simulink model "AC_Quadcopter_Simulation_Lyapnov_Hamilton_ITAE"  (R2015b)
settings: Solver=ode23  StartTime=0.0  StopTime=10  RelTol=1e-3
settings Model: Creator=HKJ  LastModifiedBy=HL

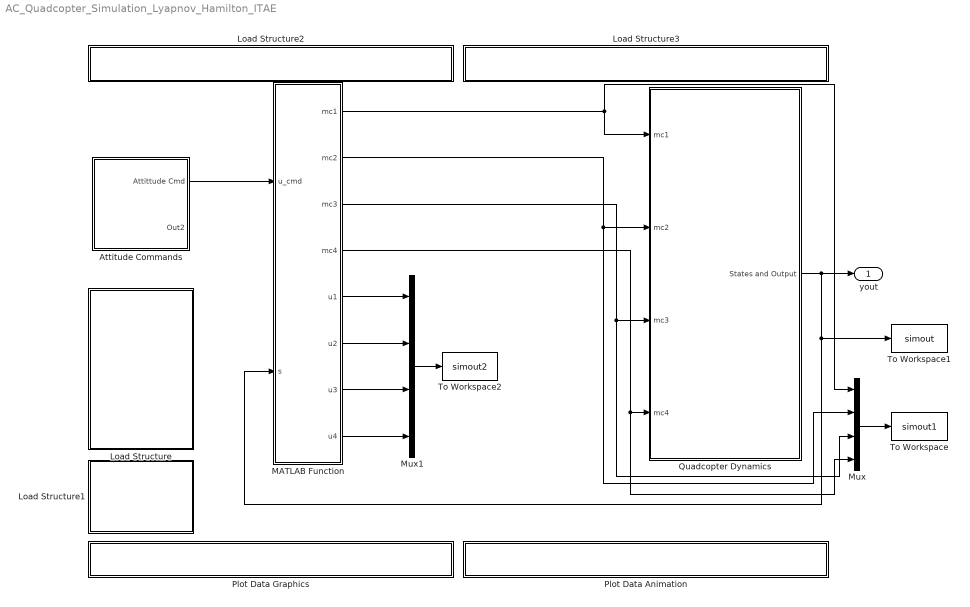
== system AC_Quadcopter_Simulation_Lyapnov_Hamilton_ITAE ==
  Attitude Commands : Subsystem
  Load Structure : Subsystem
      settings: OpenFcn=|
      | uiopen('load')
      | if (exist('IC')==1 && exist('quadModel')==1)
      | set_param(bdroot, 'SimulationCommand', 'update')
      | end
      mask Display: fprintf('LOAD:\nQuadcopter\nModel Or\nInitial\nConditions');
  Load Structure1 : Subsystem
      settings: OpenFcn=|
      | if (exist('IC')==1 && exist('quadModel')==1 && exist('yout') && exist('tout'))
      | saveSimResults()
      | else
      | msgbox('No Data To Save!')
      | end
      mask Display: fprintf('SAVE:\nSimulation\nResults');
  Load Structure2 : Subsystem
      settings: OpenFcn=|
      | if exist('GUI_Modeling') == 2,
      | run('GUI_Modeling')
      | 
      | else
      | 
      | msgbox('The desired GUI must be first added to MATLABs path.')
      | 
      | end
      mask Display: fprintf('OPEN GUI: Build New \n Model');
  Load Structure3 : Subsystem
      settings: OpenFcn=|
      | if exist('GUI_IC') == 2,
      | run('GUI_IC')
      | 
      | else
      | 
      | msgbox('The desired GUI must be first added to MATLABs path.')
      | 
      | end
      mask Display: fprintf('OPEN GUI: Create Initial \n Conditions');
  MATLAB Function : MATLAB Function  TreatAsAtomicUnit=on
  Mux : Mux
  Mux1 : Mux
  Plot Data Animation : Subsystem
      settings: OpenFcn=|
      | if exist('QuadAnim4') == 2,
      |     if exist('yout')
      | 	run('QuadAnim4');
      |     else
      |     msgbox('Simulation must be run before data can be plotted.');
      |     end
      | else                                                                          msgbox('The desired GUI must be first added to MATLABs path.')
      | end
      mask Display: fprintf('OPEN GUI: Flight Animation')
  Plot Data Graphics : Subsystem
      settings: OpenFcn=|
      | if exist('yout')
      | yout = evalin('base', 'yout');
      | tout = evalin('base', 'tout');
      | quadPlots(yout, tout)
      | else
      | msgbox('Simulation must be run before data can be plotted.')
      | end
      mask Display: fprintf('OPEN PLOT: State Data')
  Quadcopter Dynamics : Subsystem
  To Workspace : ToWorkspace  VariableName=simout1  SampleTime=-1
      settings: Save2DSignal=2-D array (concatenate along first dimension)
  To Workspace1 : ToWorkspace  VariableName=simout  SampleTime=-1
      settings: Save2DSignal=2-D array (concatenate along first dimension)
  To Workspace2 : ToWorkspace  VariableName=simout2  SampleTime=-1
      settings: Save2DSignal=2-D array (concatenate along first dimension)
  yout : Outport
  wires:
  Quadcopter Dynamics/1(States and Output) -> To Workspace1/1, MATLAB Function/2(s), yout/1
  MATLAB Function/1(mc1) -> Quadcopter Dynamics/1(mc1), Mux/1
  MATLAB Function/2(mc2) -> Quadcopter Dynamics/2(mc2), Mux/2
  MATLAB Function/3(mc3) -> Quadcopter Dynamics/3(mc3), Mux/3
  MATLAB Function/4(mc4) -> Quadcopter Dynamics/4(mc4), Mux/4
  Attitude Commands/1(Attittude Cmd) -> MATLAB Function/1(u_cmd)
  Mux/1 -> To Workspace/1
  Mux1/1 -> To Workspace2/1
  MATLAB Function/5(u1) -> Mux1/1
  MATLAB Function/6(u2) -> Mux1/2
  MATLAB Function/7(u3) -> Mux1/3
  MATLAB Function/8(u4) -> Mux1/4

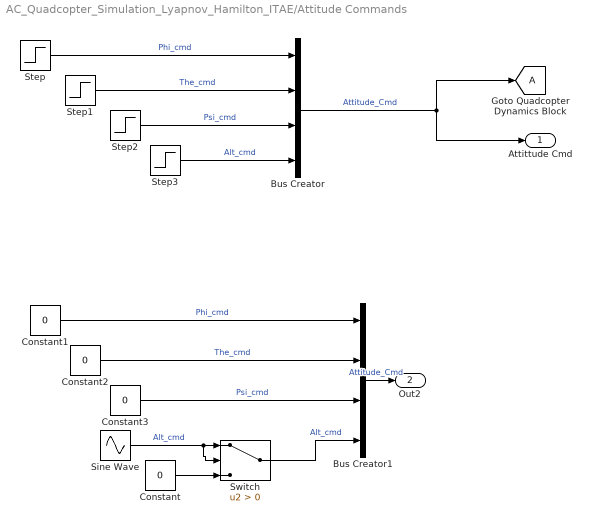
== system AC_Quadcopter_Simulation_Lyapnov_Hamilton_ITAE/Attitude Commands ==
  Bus Creator : BusCreator  Inputs=4
  Bus Creator1 : BusCreator  Inputs=4
  Constant{,1..3} (4 alike) : Constant  Value=0
  Sine Wave : Sin  Amplitude=10*0.3048  Frequency=0.2*3.1415
  Step : Step  Time=0  After=-15*pi/180  SampleTime=0
  Step1 : Step  Time=0  After=15*pi/180  SampleTime=0
  Step2 : Step  Time=0  After=15*pi/180  SampleTime=0
  Step3 : Step  Time=0  After=-1  SampleTime=0
  Switch : Switch  Criteria=u2 > Threshold
  Attittude Cmd : Outport
  Out2 : Outport  Port=2
  tag scope: A=global
  wires:
  Bus Creator/1 -> Attittude Cmd/1, [A]  "Attitude_Cmd"
  Step3/1 -> Bus Creator/4  "Alt_cmd"
  Step2/1 -> Bus Creator/3  "Psi_cmd"
  Step1/1 -> Bus Creator/2  "The_cmd"
  Step/1 -> Bus Creator/1  "Phi_cmd"
  Constant3/1 -> Bus Creator1/3  "Psi_cmd"
  Constant2/1 -> Bus Creator1/2  "The_cmd"
  Constant1/1 -> Bus Creator1/1  "Phi_cmd"
  Sine Wave/1 -> Switch/2, Switch/1  "Alt_cmd"
  Switch/1 -> Bus Creator1/4  "Alt_cmd"
  Constant/1 -> Switch/3
  Bus Creator1/1 -> Out2/1  "Attitude_Cmd"

== system AC_Quadcopter_Simulation_Lyapnov_Hamilton_ITAE/Load Structure ==

== system AC_Quadcopter_Simulation_Lyapnov_Hamilton_ITAE/Load Structure1 ==

== system AC_Quadcopter_Simulation_Lyapnov_Hamilton_ITAE/Load Structure2 ==

== system AC_Quadcopter_Simulation_Lyapnov_Hamilton_ITAE/Load Structure3 ==

== system AC_Quadcopter_Simulation_Lyapnov_Hamilton_ITAE/Plot Data Animation ==

== system AC_Quadcopter_Simulation_Lyapnov_Hamilton_ITAE/Plot Data Graphics ==

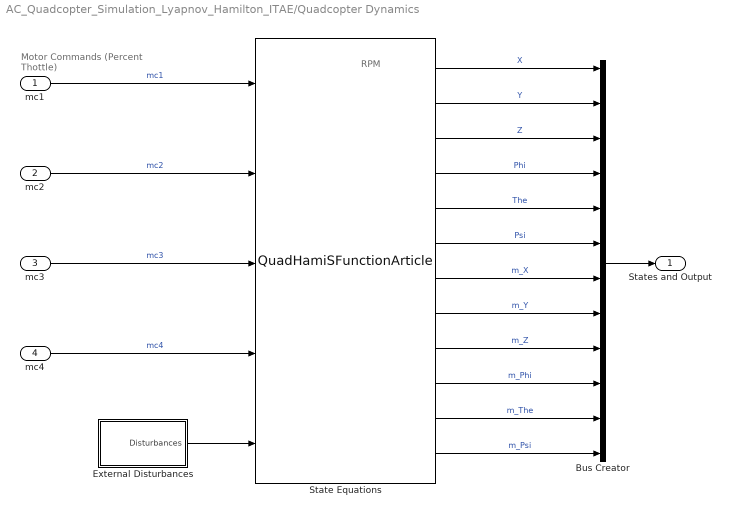
== system AC_Quadcopter_Simulation_Lyapnov_Hamilton_ITAE/Quadcopter Dynamics ==
  note: Motor Commands
      | (Percent Thottle)
  note: RPM
  mc1 : Inport
  mc2 : Inport  Port=2
  mc3 : Inport  Port=3
  mc4 : Inport  Port=4
  Bus Creator : BusCreator  Inputs='X','Y','Z','Phi','The','Psi','m_X','m_Y','m_Z','m_Phi','m_The','m_Psi'
  External Disturbances : Subsystem
  State Equations : M-S-Function  FunctionName=QuadHamiSFunctionArticle  Parameters=quadModel, IC
      mask Display:
      | port_label('input', 1, 'RPM1')
      | port_label('input', 2, 'RPM2')
      | port_label('input', 3, 'RPM3')
      | port_label('input', 4, 'RPM4')
      | port_label('input', 5, 'Disturbances')
      | port_label('output', 1, 'X')
      | port_label('output', 2, 'Y')
      | port_label('output', 3, 'Z')
      | port_label('output', 4, 'Phi')
      | port_label('output', 5, 'The')
      | port_label('output', 6, 'Psi')
      | port_label('output', 7, 'm_X')
      | port_label('output', 8, 'm_Y')
      | port_label('output', 9, 'm_Z')
      | port_label('output', 10, 'm_Phi')
      | port_label('output', 11, 'm_The')
      | port_label('output', 12, 'm_Psi')
  States and Output : Outport
  wires:
  mc1/1 -> State Equations/1  "mc1"
  mc2/1 -> State Equations/2  "mc2"
  mc3/1 -> State Equations/3  "mc3"
  mc4/1 -> State Equations/4  "mc4"
  State Equations/1 -> Bus Creator/1  "X"
  State Equations/2 -> Bus Creator/2  "Y"
  State Equations/3 -> Bus Creator/3  "Z"
  State Equations/4 -> Bus Creator/4  "Phi"
  State Equations/5 -> Bus Creator/5  "The"
  State Equations/6 -> Bus Creator/6  "Psi"
  State Equations/7 -> Bus Creator/7  "m_X"
  State Equations/8 -> Bus Creator/8  "m_Y"
  State Equations/9 -> Bus Creator/9  "m_Z"
  State Equations/10 -> Bus Creator/10  "m_Phi"
  State Equations/11 -> Bus Creator/11  "m_The"
  State Equations/12 -> Bus Creator/12  "m_Psi"
  Bus Creator/1 -> States and Output/1
  External Disturbances/1("Disturbances ") -> State Equations/5

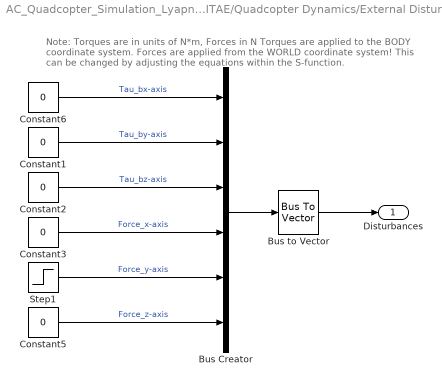
== system AC_Quadcopter_Simulation_Lyapnov_Hamilton_ITAE/Quadcopter Dynamics/External Disturbances ==
  note: Note: Torques are in units of N*m, Forces in N
      | Torques are applied to the BODY coordinate system.
      | Forces are applied from the WORLD coordinate system!
      | This can be changed by adjusting the equations within the S-function.
  Bus Creator : BusCreator  Inputs=6
  Bus to Vector : BusToVector
  Constant{1..3,5..6} (5 alike) : Constant  Value=0
  Step1 : Step  After=0  SampleTime=0
  "Disturbances " : Outport
  wires:
  Bus to Vector/1 -> "Disturbances "/1
  Bus Creator/1 -> Bus to Vector/1
  Constant6/1 -> Bus Creator/1  "Tau_bx-axis"
  Constant1/1 -> Bus Creator/2  "Tau_by-axis"
  Constant2/1 -> Bus Creator/3  "Tau_bz-axis"
  Constant3/1 -> Bus Creator/4  "Force_x-axis"
  Step1/1 -> Bus Creator/5  "Force_y-axis"
  Constant5/1 -> Bus Creator/6  "Force_z-axis"

== matlab function AC_Quadcopter_Simulation_Lyapnov_Hamilton_ITAE/MATLAB Function ==
  data: u_cmd input; mc1 output; s input; mc2 output; mc3 output; mc4 output; u1 output; u2 output; u3 output; u4 output
function [mc1,mc2,mc3,mc4,u1,u2,u3,u4] = fcn(u_cmd,s)
%自己设计的控制器
k1 = 3.9210;
k2 = 8;
k3 = 3.9210;
k4 = 8;
k5 = 2.6557;
k6 = 2.5;

k11 = 2;
k12 = 2;
% k1 = 1;
% k2 = 50;
% k3 = 1;
% k4 = 50;
% k5 = 1;
% k6 = 50;
% 
% k11 = 1.5;
% k12 = 1.5;
Ix = 0.0094999;Iy=0.0094999;Iz=0.018576;
I = [Ix,0,0;0,Iy,0;0,0,Iz];
m=1.023;g=9.81;
% L=0.185738;%z这个值有问题
ct=1.4865e-07;
cq=2.925e-09;
ctl = 3.30374625e-08;

phi_cmd = u_cmd(1);
the_cmd = u_cmd(2);
psi_cmd = u_cmd(3);
alt_cmd = u_cmd(4);
z = s(3);
Phi = s(4);The = s(5);Psi = s(6);
m_z = s(9);
m_Phi = s(10);m_The = s(11);m_Psi = s(12);

dPhi = (Iy*Iz+(Ix-Iz)*Iy*sin(The)^2-(Iy-Iz)*Ix*sin(Phi)^2*sin(The)^2)*m_Phi/(Ix*Iy*Iz*cos(The)^2)+...
       (-(Iy-Iz)*cos(Phi)*sin(Phi)*sin(The)*m_The)/(Iy*Iz*cos(The))+...
       (Iy*cos(Phi)^2+Iz*sin(Phi)^2)*sin(The)*m_Psi/(Iy*Iz*cos(The)^2);
dThe = -(Iy-Iz)*cos(Phi)*sin(Phi)*sin(The)*m_Phi/(Iy*Iz*cos(The))+...
       (Iy*sin(Phi)^2+Iz*cos(Phi)^2)*m_The/(Iy*Iz)+...
       (-(Iy-Iz)*cos(Phi)*sin(Phi))*m_Psi/(Iy*Iz*cos(The));
dPsi = (Iy*cos(Phi)^2+Iz*sin(Phi)^2)*sin(The)*m_Phi/(Iy*Iz*cos(The)^2)+...
       (-(Iy-Iz)*cos(Phi)*sin(Phi))*m_The/(Iy*Iz*cos(The))+...
       (Iy*cos(Phi)^2+Iz*sin(Phi)^2)*m_Psi/(Iy*Iz*cos(The)^2);

g1 = (Iy*Iz+(Ix-Iz)*Iy*sin(The)^2-(Iy-Iz)*Ix*sin(Phi)^2*sin(The)^2)/(Ix*Iy*Iz*cos(The)^2);
g2 = (Iy*sin(Phi)^2+Iz*cos(Phi)^2)/(Iy*Iz);
g3 = (Iy*cos(Phi)^2+Iz*sin(Phi)^2)/(Iy*Iz*cos(The)^2);

g12 = -(Iy-Iz)*cos(Phi)*sin(Phi)*sin(The)/(Iy*Iz*cos(The));
g13 = (Iy*cos(Phi)^2+Iz*sin(Phi)^2)*sin(The)/(Iy*Iz*cos(The)^2);
g23 = -(Iy-Iz)*cos(Phi)*sin(Phi)/(Iy*Iz*cos(The));

J = [g1,g12,g13;g12,g2,g23;g13,g23,g3];

f1 = -(Iy-Iz)*(dThe^2*sin(Phi)*cos(Phi)-dThe*dPsi*cos(2*Phi)*cos(The)-dPsi^2*sin(Phi)*cos(Phi)*cos(The)^2);
f2 = (Ix-Iy*sin(Phi)^2-Iz*cos(Phi)^2)*dPsi^2*sin(The)*cos(The)-(Iy-Iz)*dThe*dPsi*sin(Phi)*cos(Phi)*sin(The)-dPhi*dPsi*Ix*cos(The);

e11 = z-alt_cmd;
e12 = m_z/m+k11*e11;
u1 = (-m*g+m*((k11^2-1)*e11-(k11+k12)*e12))/(cos(phi_cmd)*cos(the_cmd));

e1 = Phi-phi_cmd;
e2 = m_Phi/Ix+k1*e1;
e3 = The-the_cmd;
e4 = m_The/Iy+k3*e3;
e5 = Psi-psi_cmd;
e6 = m_Psi/Iz+k5*e5;

K_eta = [k1,0,0;0,k3,0;0,0,k5];
K_peta = [k2,0,0;0,k4,0;0,0,k6];
e_eta = [e1;e3;e5];
e_peta = [e2;e4;e6];
tau_p=I*((K_eta*J*I*K_eta-J*I)*e_eta-(K_eta+K_peta)*J*I*e_peta)-[f1;f2;0];
u2 = tau_p(1);
u3 = tau_p(2);
u4 = tau_p(3);
% u2 = -f1+(-(k1*g1*Ix+k2)*e2+(g1*Ix*k1^2-g1*Ix)*e1)*Ix;
% u3 = -f2+(-(k3*g2*Iy+k4)*e4+(g2*Iy*k3^2-g2*Iy)*e3)*Iy;
% u4 =(-(k5*g3*Iz+k6)*e6+(g3*Iz*k5^2-g3*Iz)*e5)*Iz;

mc1 = sqrt((-u1/ct+u4/cq)*0.25+u3/ctl*0.5);
mc2 = sqrt((-u1/ct-u4/cq)*0.25+u2/ctl*0.5);
mc3 = sqrt((-u1/ct+u4/cq)*0.25-u3/ctl*0.5);
mc4 = sqrt((-u1/ct-u4/cq)*0.25-u2/ctl*0.5);
